simulink model "Homing_control"  (R2019b)
settings: Solver=FixedStepAuto  StartTime=0.0  StopTime=inf  FixedStep=0.01  RelTol=1e-3
undefined symbols (not defined in the file or in its folder): canChannel
libraries: canmsglib x13, simulink x7, canlib x3, sldrtlib x1
settings Model: Creator=Mohsen  LastModifiedBy=Mohsen
settings DataIOCC: ReturnWorkspaceOutputs=off
settings DebuggingCC: ArithmeticOperatorsInVariantConditions=warning
settings SFSimCC: SimUseLocalCustomCode=off  CustomCodeUndefinedFunction=UseInterfaceOnly
settings RTWCC: Description=Simulink Desktop Real-Time  SystemTargetFile=sldrt.tlc  TemplateMakefile=sldrt.tmf  RTWUseLocalCustomCode=off  RTWCompilerOptimization=on
settings CodeAppCC: MaxIdLength=95
settings TargetCC: TargetPreCompLibLocation=C:\Program Files\MATLAB\R2018b\toolbox\sldrt\lib\win64  TargetLangStandard=C99 (ISO)  GeneratePreprocessorConditionals=Use local settings  SupportVariableSizeSignals=on  PreserveStateflowLocalDataDimensions=off

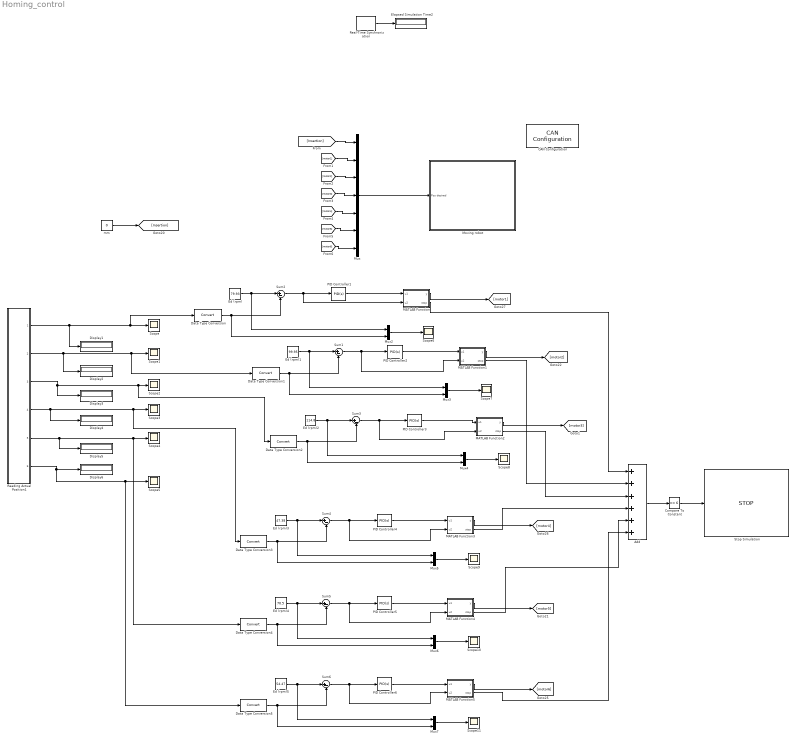
== system Homing_control ==
  Add : Sum  Inputs=++++++
  CAN Configuration : canlib/CAN Configuration  BlockHandle=3.0001  Device=Kvaser USBcan Light 1 (Channel 1)  DeviceMenu=Kvaser USBcan Light 1 (Channel 1)  ObjConstructor=canChannel('Kvaser', 'USBcan Light 1', 1)  BusSpeed=500000  EnableBitParameters=off  SJW=1  TSEG1=4  TSEG2=3  NSamples=1  AckMode=Normal
      settings: SourceProductName=Vehicle Network Toolbox  SourceProductBaseCode=VN
  Compare To Constant : simulink/Logic and Bit Operations/Compare To Constant  relop===  const=6  OutDataTypeStr=boolean
  Data Type Conversion{,1..5} (6 alike) : DataTypeConversion
  Display{1..6} (6 alike) : Display
  Ed (rpm) : Constant  Value=79.93
  Ed (rpm)1 : Constant  Value=99.95
  Ed (rpm)2 : Constant  Value=114.8
  Ed (rpm)3 : Constant  Value=47.38
  Ed (rpm)4 : Constant  Value=70.5
  Ed (rpm)5 : Constant  Value=54.47
  Elapsed Simulation Time2 : Display
      settings: Decimation=2
  MATLAB Function : MATLAB Function  TreatAsAtomicUnit=on
  MATLAB Function1 : MATLAB Function  TreatAsAtomicUnit=on
  MATLAB Function2 : MATLAB Function  TreatAsAtomicUnit=on
  MATLAB Function3 : MATLAB Function  TreatAsAtomicUnit=on
  MATLAB Function4 : MATLAB Function  TreatAsAtomicUnit=on
  MATLAB Function5 : MATLAB Function  TreatAsAtomicUnit=on
  Moving robot : Subsystem
  Mux : Mux  Inputs=7
  Mux{2..7} (6 alike) : Mux  Inputs=2
  PID Controller{1..6} (6 alike) : simulink/Continuous/PID Controller  Controller=PID  Form=Parallel  TimeDomain=Continuous-time  SampleTime=-1  IntegratorMethod=Forward Euler  FilterMethod=Forward Euler  ControllerParametersSource=internal  P=200  I=5  D=1  UseFilter=on  N=100  TunerSelectOption=Frequency Response Based  InitialConditionSource=internal  InitialConditionForIntegrator=0  InitialConditionForFilter=0  DifferentiatorICPrevScaledInput=0  ExternalReset=none  TrackingMode=off  Kt=1  LimitOutput=off  UpperSaturationLimit=inf  LowerSaturationLimit=-inf  LinearizeAsGain=on  AntiWindupMode=none  Kb=1  POutMin=[]  POutMax=[]  IOutMin=[]  IOutMax=[]  DOutMin=[]  DOutMax=[]  NOutMin=[]  NOutMax=[]  SumOutMin=[]  SumOutMax=[]  SaturationOutMin=[]  SaturationOutMax=[]  PParamMin=[]  PParamMax=[]  IParamMin=[]  IParamMax=[]  DParamMin=[]  DParamMax=[]  NParamMin=[]  NParamMax=[]  KbParamMin=[]  KbParamMax=[]  KtParamMin=[]  KtParamMax=[]  KbOutMin=[]  KbOutMax=[]  KtOutMin=[]  KtOutMax=[]  IntegratorOutMin=[]  IntegratorOutMax=[]  FilterOutMin=[]  FilterOutMax=[]  SumI1OutMin=[]  SumI1OutMax=[]  SumI2OutMin=[]  SumI2OutMax=[]  SumI3OutMin=[]  SumI3OutMax=[]  SumI4OutMin=[]  SumI4OutMax=[]  SumDOutMin=[]  SumDOutMax=[]  DifferentiatorOutMin=[]  DifferentiatorOutMax=[]  FilterDiffOutCoefMin=[]  FilterDiffOutCoefMax=[]  ReciprocalOutMin=[]  ReciprocalOutMax=[]  SumDenOutMin=[]  SumDenOutMax=[]  SumNumOutMin=[]  SumNumOutMax=[]  DivideOutMin=[]  DivideOutMax=[]  IntegratorContinuousStateAttributes=''  IntegratorStateMustResolveToSignalObject=off  IntegratorRTWStateStorageClass=Auto  FilterContinuousStateAttributes=''  FilterStateMustResolveToSignalObject=off  FilterRTWStateStorageClass=Auto  ParallelPVariant=InternalParameters  IdealPVariant=Disabled  IVariant=InternalParameters  DVariant=InternalParameters  IntegratorVariant=Continuous  SatVariant=Disabled  AWVariant=Passthrough  PCopyVariant=Disabled  TRVariant=Disabled  FdbkBlocksVariant=Forward  IdealPFdbkVariant=Disabled  SatFdbkVariant=Disabled  DerivativeFilterVariant=ContFilter  NVariant=InternalParameters  NCopyVariant=Disabled  FilterICVariant=InternalICsFilter  IntegratorICVariant=InternalICs  ExternalResetVariant=Disabled  TRSumVariant=Passthrough  SumFdbkVariant=Disabled  SumVariant=Sum_PID
  Reading Actual Position1 : Subsystem
  Real-Time Synchronization : sldrtlib/Real-Time Synchronization  SampleTime=-1  MaxMissedTicks=inf  ShowMissedTicks=on  YieldWhenWaiting=off
  Scope{,1..11} (12 alike) : Scope
  Stop Simulation : Stop
  Sum{1..6} (6 alike) : Sum  Inputs=|+-
  mm : Constant  Value=0
  wires:
  Mux/1 -> Moving robot/1(Pos desired)
  [motor6] -> Mux/7
  [motor5] -> Mux/6
  [motor4] -> Mux/5
  [motor3] -> Mux/4
  [motor2] -> Mux/3
  [motor1] -> Mux/2
  [Insertion] -> Mux/1
  mm/1 -> [Insertion]
  Real-Time Synchronization/1 -> Elapsed Simulation Time2/1
  Ed (rpm)/1 -> Mux2/1, Sum2/1
  Sum2/1 -> MATLAB Function/2(u2), PID Controller1/1
  Mux2/1 -> Scope6/1
  Reading Actual Position1/1(1) -> Data Type Conversion/1, Scope/1, Display1/1
  Data Type Conversion/1 -> Mux2/2, Sum2/2
  PID Controller1/1 -> MATLAB Function/1(u1)
  MATLAB Function1/1(y) -> [motor2]
  Mux3/1 -> Scope7/1
  Ed (rpm)1/1 -> Mux3/1, Sum1/1
  Reading Actual Position1/2(2) -> Display2/1, Data Type Conversion1/1, Scope1/1
  Sum1/1 -> PID Controller2/1, MATLAB Function1/2(u2)
  Data Type Conversion1/1 -> Mux3/2, Sum1/2
  PID Controller2/1 -> MATLAB Function1/1(u1)
  MATLAB Function2/1(y) -> [motor3]
  Mux4/1 -> Scope8/1
  Ed (rpm)2/1 -> Mux4/1, Sum3/1
  Reading Actual Position1/3(3) -> Data Type Conversion2/1, Scope2/1, Display3/1
  Sum3/1 -> MATLAB Function2/2(u2), PID Controller3/1
  Data Type Conversion2/1 -> Mux4/2, Sum3/2
  PID Controller3/1 -> MATLAB Function2/1(u1)
  MATLAB Function3/1(y) -> [motor4]
  Mux5/1 -> Scope9/1
  Ed (rpm)3/1 -> Mux5/1, Sum4/1
  Reading Actual Position1/4(4) -> Data Type Conversion3/1, Scope3/1, Display4/1
  Sum4/1 -> MATLAB Function3/2(u2), PID Controller4/1
  Data Type Conversion3/1 -> Mux5/2, Sum4/2
  PID Controller4/1 -> MATLAB Function3/1(u1)
  MATLAB Function4/1(y) -> [motor5]
  Mux6/1 -> Scope10/1
  Ed (rpm)4/1 -> Mux6/1, Sum5/1
  Reading Actual Position1/5(5) -> Display5/1, Data Type Conversion4/1, Scope4/1
  Sum5/1 -> MATLAB Function4/2(u2), PID Controller5/1
  Data Type Conversion4/1 -> Mux6/2, Sum5/2
  PID Controller5/1 -> MATLAB Function4/1(u1)
  MATLAB Function5/1(y) -> [motor6]
  Mux7/1 -> Scope11/1
  Ed (rpm)5/1 -> Mux7/1, Sum6/1
  Reading Actual Position1/6(6) -> Data Type Conversion5/1, Scope5/1, Display6/1
  Sum6/1 -> MATLAB Function5/2(u2), PID Controller6/1
  Data Type Conversion5/1 -> Mux7/2, Sum6/2
  PID Controller6/1 -> MATLAB Function5/1(u1)
  MATLAB Function/1(y) -> [motor1]
  Add/1 -> Compare To Constant/1
  MATLAB Function/2(stop) -> Add/1
  MATLAB Function1/2(stop) -> Add/2
  MATLAB Function2/2(stop) -> Add/3
  MATLAB Function3/2(stop) -> Add/4
  MATLAB Function4/2(stop) -> Add/5
  MATLAB Function5/2(stop) -> Add/6
  Compare To Constant/1 -> Stop Simulation/1

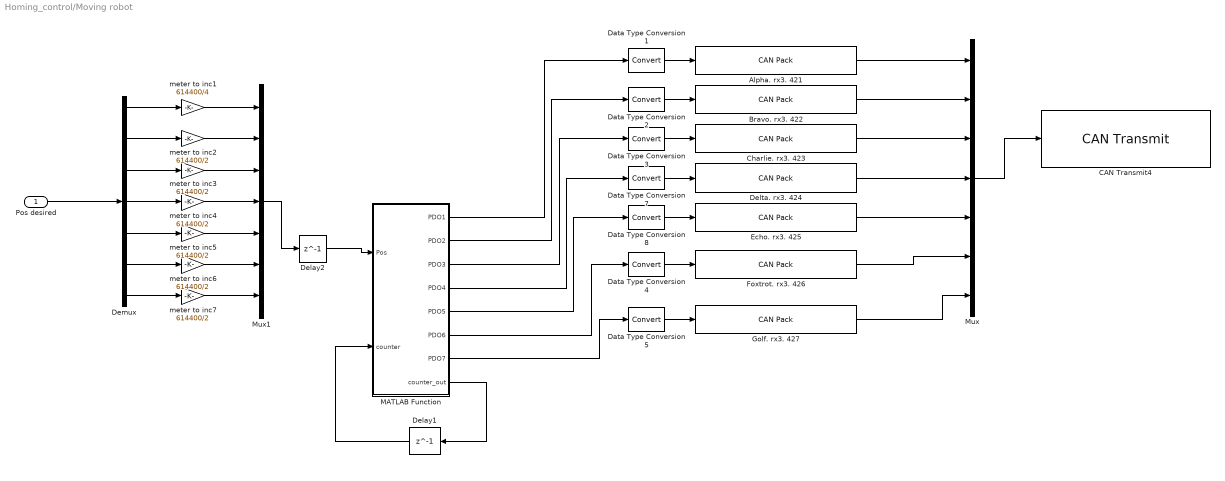
== system Homing_control/Moving robot ==
  Pos desired : Inport
  Alpha. rx3. 421 : canmsglib/CAN Pack  MsgList=(none)  MsgName=Alpha  MsgIDType=Standard (11-bit identifier)  MsgIdentifier=1057  MsgLength=8  Remote=off  ApplyMinMax=off  BusOutput=off  SignalInfo={ 'clear', '0', '64', 'LE', 'unsigned', 'Standard', '0', '1', '0', '-Inf', 'Inf' }
      settings: SourceProductName=Simulink Real-Time  SourceProductBaseCode=XP  DataFormat=raw data
  Bravo. rx3. 422 : canmsglib/CAN Pack  MsgList=(none)  MsgName=Bravo  MsgIDType=Standard (11-bit identifier)  MsgIdentifier=1058  MsgLength=8  Remote=off  ApplyMinMax=off  BusOutput=off  SignalInfo={ 'clear', '0', '64', 'LE', 'unsigned', 'Standard', '0', '1', '0', '-Inf', 'Inf' }
      settings: SourceProductName=Simulink Real-Time  SourceProductBaseCode=XP  DataFormat=raw data
  CAN Transmit4 : canlib/CAN Transmit  BlockHandle=1540.0004  Device=Kvaser USBcan Light 1 (Channel 1)  DeviceMenu=Kvaser USBcan Light 1 (Channel 1)  ObjConstructor=canChannel('Kvaser', 'USBcan Light 1', 1)  EnablePeriodicTransmit=off  MessagePeriod=0.500
      settings: SourceProductName=Vehicle Network Toolbox  SourceProductBaseCode=VN
  Charlie. rx3. 423 : canmsglib/CAN Pack  MsgList=(none)  MsgName=Charlie  MsgIDType=Standard (11-bit identifier)  MsgIdentifier=1059  MsgLength=8  Remote=off  ApplyMinMax=off  BusOutput=off  SignalInfo={ 'clear', '0', '64', 'LE', 'unsigned', 'Standard', '0', '1', '0', '-Inf', 'Inf' }
      settings: SourceProductName=Simulink Real-Time  SourceProductBaseCode=XP  DataFormat=raw data
  Data Type Conversion{1..5,7..8} (7 alike) : DataTypeConversion
  Delay1 : Delay  DelayLength=1  InitialCondition=0
  Delay2 : Delay  DelayLength=1  InitialCondition=[ 0 0 0 0 0 0 0]
  Delta. rx3. 424 : canmsglib/CAN Pack  MsgList=(none)  MsgName=Delta  MsgIDType=Standard (11-bit identifier)  MsgIdentifier=1060  MsgLength=8  Remote=off  ApplyMinMax=off  BusOutput=off  SignalInfo={ 'clear', '0', '64', 'LE', 'unsigned', 'Standard', '0', '1', '0', '-Inf', 'Inf' }
      settings: SourceProductName=Simulink Real-Time  SourceProductBaseCode=XP  DataFormat=raw data
  Demux : Demux  Outputs=7
  Echo. rx3. 425 : canmsglib/CAN Pack  MsgList=(none)  MsgName=Echo  MsgIDType=Standard (11-bit identifier)  MsgIdentifier=1061  MsgLength=8  Remote=off  ApplyMinMax=off  BusOutput=off  SignalInfo={ 'clear', '0', '64', 'LE', 'unsigned', 'Standard', '0', '1', '0', '-Inf', 'Inf' }
      settings: SourceProductName=Simulink Real-Time  SourceProductBaseCode=XP  DataFormat=raw data
  Foxtrot. rx3. 426 : canmsglib/CAN Pack  MsgList=(none)  MsgName=Foxtrot  MsgIDType=Standard (11-bit identifier)  MsgIdentifier=1062  MsgLength=8  Remote=off  ApplyMinMax=off  BusOutput=off  SignalInfo={ 'clear', '0', '64', 'LE', 'unsigned', 'Standard', '0', '1', '0', '-Inf', 'Inf' }
      settings: SourceProductName=Simulink Real-Time  SourceProductBaseCode=XP  DataFormat=raw data
  Golf. rx3. 427 : canmsglib/CAN Pack  MsgList=(none)  MsgName=Golf  MsgIDType=Standard (11-bit identifier)  MsgIdentifier=1063  MsgLength=8  Remote=off  ApplyMinMax=off  BusOutput=off  SignalInfo={ 'clear', '0', '64', 'LE', 'unsigned', 'Standard', '0', '1', '0', '-Inf', 'Inf' }
      settings: SourceProductName=Simulink Real-Time  SourceProductBaseCode=XP  DataFormat=raw data
  MATLAB Function : MATLAB Function  TreatAsAtomicUnit=on
  Mux : Mux  Inputs=7
  Mux1 : Mux  Inputs=7
  meter to inc1 : Gain  Gain=614400/4
  meter to inc{2..7} (6 alike) : Gain  Gain=614400/2
  wires:
  Data Type Conversion1/1 -> Alpha. rx3. 421/1
  MATLAB Function/8(counter_out) -> Delay1/1
  Delay1/1 -> MATLAB Function/2(counter)
  Mux/1 -> CAN Transmit4/1
  Mux1/1 -> Delay2/1
  Delay2/1 -> MATLAB Function/1(Pos)
  Alpha. rx3. 421/1 -> Mux/1
  Pos desired/1 -> Demux/1
  Demux/7 -> meter to inc7/1
  meter to inc7/1 -> Mux1/7
  Demux/6 -> meter to inc6/1
  meter to inc6/1 -> Mux1/6
  meter to inc5/1 -> Mux1/5
  Demux/5 -> meter to inc5/1
  Demux/4 -> meter to inc4/1
  meter to inc4/1 -> Mux1/4
  meter to inc3/1 -> Mux1/3
  meter to inc2/1 -> Mux1/2
  meter to inc1/1 -> Mux1/1
  Demux/1 -> meter to inc1/1
  Demux/2 -> meter to inc2/1
  Demux/3 -> meter to inc3/1
  Data Type Conversion2/1 -> Bravo. rx3. 422/1
  Data Type Conversion3/1 -> Charlie. rx3. 423/1
  Data Type Conversion7/1 -> Delta. rx3. 424/1
  Data Type Conversion8/1 -> Echo. rx3. 425/1
  Bravo. rx3. 422/1 -> Mux/2
  Charlie. rx3. 423/1 -> Mux/3
  Delta. rx3. 424/1 -> Mux/4
  Echo. rx3. 425/1 -> Mux/5
  MATLAB Function/1(PDO1) -> Data Type Conversion1/1
  MATLAB Function/2(PDO2) -> Data Type Conversion2/1
  MATLAB Function/3(PDO3) -> Data Type Conversion3/1
  MATLAB Function/4(PDO4) -> Data Type Conversion7/1
  MATLAB Function/5(PDO5) -> Data Type Conversion8/1
  Data Type Conversion4/1 -> Foxtrot. rx3. 426/1
  Data Type Conversion5/1 -> Golf. rx3. 427/1
  MATLAB Function/6(PDO6) -> Data Type Conversion4/1
  MATLAB Function/7(PDO7) -> Data Type Conversion5/1
  Foxtrot. rx3. 426/1 -> Mux/6
  Golf. rx3. 427/1 -> Mux/7

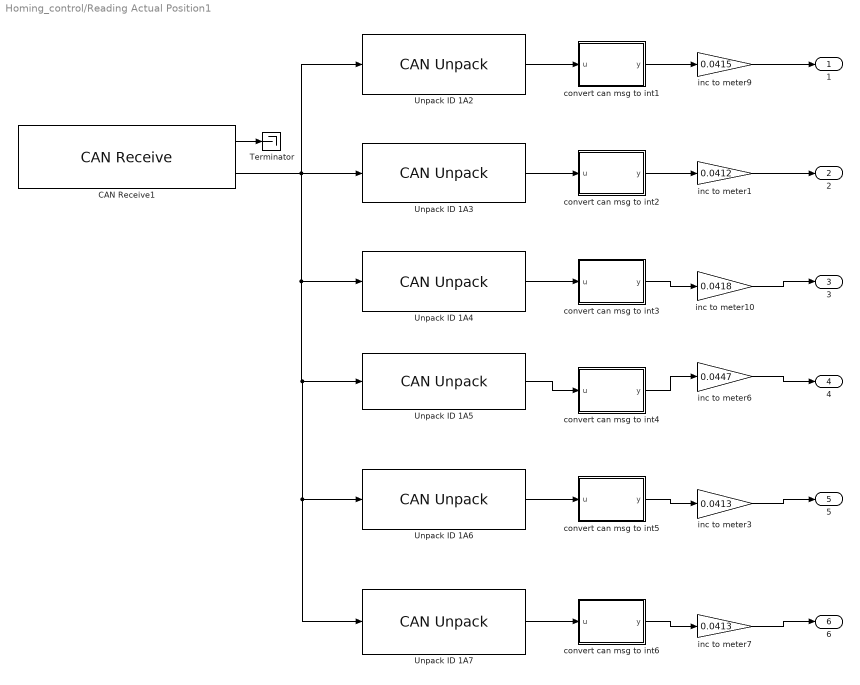
== system Homing_control/Reading Actual Position1 ==
  CAN Receive1 : canlib/CAN Receive  BlockHandle=1635.0002  Device=Kvaser USBcan Light 1 (Channel 1)  DeviceMenu=Kvaser USBcan Light 1 (Channel 1)  ObjConstructor=canChannel('Kvaser', 'USBcan Light 1', 1)  EnableStandardIDsFilter=off  StdIDsCombo=Allow only  StandardIDs=[418 419 420 421 422 423]  EnableExtendedIDsFilter=off  ExtIDsCombo=Allow all  ExtendedIDs=0  SampleTime=-1  MsgsPerTimestep=all  InternalFilterUpdateStatus=on  BusOutput=off
      settings: SourceProductName=Vehicle Network Toolbox  SourceProductBaseCode=VN
  Terminator : Terminator
  Unpack ID 1A2 : canmsglib/CAN Unpack  MsgList=(none)  MsgName=CAN Msg  MsgIDType=Standard (11-bit identifier)  MsgIdentifier=418  MsgLength=2  SignalInfo={ 'Counter', '8', '16', 'LE', 'unsigned', 'Standard', '0', '1', '0', '-Inf', 'Inf' }  IDPort=off  TimestampPort=off  ErrorPort=off  RemotePort=off  LengthPort=off  StatusPort=off  ApplyMinMax=off
      settings: SourceProductName=Simulink Real-Time  SourceProductBaseCode=XP  DataFormat=raw data
  Unpack ID 1A3 : canmsglib/CAN Unpack  MsgList=(none)  MsgName=CAN Msg  MsgIDType=Standard (11-bit identifier)  MsgIdentifier=419  MsgLength=2  SignalInfo={ 'Counter', '8', '16', 'LE', 'unsigned', 'Standard', '0', '1', '0', '-Inf', 'Inf' }  IDPort=off  TimestampPort=off  ErrorPort=off  RemotePort=off  LengthPort=off  StatusPort=off  ApplyMinMax=off
      settings: SourceProductName=Simulink Real-Time  SourceProductBaseCode=XP  DataFormat=raw data
  Unpack ID 1A4 : canmsglib/CAN Unpack  MsgList=(none)  MsgName=CAN Msg  MsgIDType=Standard (11-bit identifier)  MsgIdentifier=420  MsgLength=2  SignalInfo={ 'Counter', '8', '16', 'LE', 'unsigned', 'Standard', '0', '1', '0', '-Inf', 'Inf' }  IDPort=off  TimestampPort=off  ErrorPort=off  RemotePort=off  LengthPort=off  StatusPort=off  ApplyMinMax=off
      settings: SourceProductName=Simulink Real-Time  SourceProductBaseCode=XP  DataFormat=raw data
  Unpack ID 1A5 : canmsglib/CAN Unpack  MsgList=(none)  MsgName=CAN Msg  MsgIDType=Standard (11-bit identifier)  MsgIdentifier=421  MsgLength=2  SignalInfo={ 'Counter', '8', '16', 'LE', 'unsigned', 'Standard', '0', '1', '0', '-Inf', 'Inf' }  IDPort=off  TimestampPort=off  ErrorPort=off  RemotePort=off  LengthPort=off  StatusPort=off  ApplyMinMax=off
      settings: SourceProductName=Simulink Real-Time  SourceProductBaseCode=XP  DataFormat=raw data
  Unpack ID 1A6 : canmsglib/CAN Unpack  MsgList=(none)  MsgName=CAN Msg  MsgIDType=Standard (11-bit identifier)  MsgIdentifier=422  MsgLength=2  SignalInfo={ 'Counter', '8', '16', 'LE', 'unsigned', 'Standard', '0', '1', '0', '-Inf', 'Inf' }  IDPort=off  TimestampPort=off  ErrorPort=off  RemotePort=off  LengthPort=off  StatusPort=off  ApplyMinMax=off
      settings: SourceProductName=Simulink Real-Time  SourceProductBaseCode=XP  DataFormat=raw data
  Unpack ID 1A7 : canmsglib/CAN Unpack  MsgList=(none)  MsgName=CAN Msg  MsgIDType=Standard (11-bit identifier)  MsgIdentifier=423  MsgLength=2  SignalInfo={ 'Counter', '8', '16', 'LE', 'unsigned', 'Standard', '0', '1', '0', '-Inf', 'Inf' }  IDPort=off  TimestampPort=off  ErrorPort=off  RemotePort=off  LengthPort=off  StatusPort=off  ApplyMinMax=off
      settings: SourceProductName=Simulink Real-Time  SourceProductBaseCode=XP  DataFormat=raw data
  convert can msg to int1 : MATLAB Function  TreatAsAtomicUnit=on
  convert can msg to int2 : MATLAB Function  TreatAsAtomicUnit=on
  convert can msg to int3 : MATLAB Function  TreatAsAtomicUnit=on
  convert can msg to int4 : MATLAB Function  TreatAsAtomicUnit=on
  convert can msg to int5 : MATLAB Function  TreatAsAtomicUnit=on
  convert can msg to int6 : MATLAB Function  TreatAsAtomicUnit=on
  inc to meter1 : Gain  Gain=0.0412
  inc to meter10 : Gain  Gain=0.0418
  inc to meter3 : Gain  Gain=0.0413
  inc to meter6 : Gain  Gain=0.0447
  inc to meter7 : Gain  Gain=0.0413
  inc to meter9 : Gain  Gain=0.0415
  1 : Outport  VectorParamsAs1DForOutWhenUnconnected=off
  2 : Outport  Port=2  VectorParamsAs1DForOutWhenUnconnected=off
  3 : Outport  Port=3  VectorParamsAs1DForOutWhenUnconnected=off
  4 : Outport  Port=4  VectorParamsAs1DForOutWhenUnconnected=off
  5 : Outport  Port=5  VectorParamsAs1DForOutWhenUnconnected=off
  6 : Outport  Port=6  VectorParamsAs1DForOutWhenUnconnected=off
  wires:
  convert can msg to int3/1(y) -> inc to meter10/1
  inc to meter10/1 -> 3/1
  convert can msg to int2/1(y) -> inc to meter1/1
  Unpack ID 1A3/1 -> convert can msg to int2/1(u)
  Unpack ID 1A5/1 -> convert can msg to int4/1(u)
  inc to meter1/1 -> 2/1
  convert can msg to int5/1(y) -> inc to meter3/1
  inc to meter3/1 -> 5/1
  Unpack ID 1A7/1 -> convert can msg to int6/1(u)
  inc to meter7/1 -> 6/1
  Unpack ID 1A6/1 -> convert can msg to int5/1(u)
  Unpack ID 1A4/1 -> convert can msg to int3/1(u)
  convert can msg to int6/1(y) -> inc to meter7/1
  CAN Receive1/1 -> Terminator/1
  inc to meter6/1 -> 4/1
  convert can msg to int4/1(y) -> inc to meter6/1
  CAN Receive1/2 -> Unpack ID 1A7/1, Unpack ID 1A6/1, Unpack ID 1A5/1, Unpack ID 1A4/1, Unpack ID 1A2/1, Unpack ID 1A3/1
  Unpack ID 1A2/1 -> convert can msg to int1/1(u)
  inc to meter9/1 -> 1/1
  convert can msg to int1/1(y) -> inc to meter9/1

== matlab function Homing_control/Moving robot/MATLAB Function ==
  data: PDO1 output; PDO2 output; PDO3 output; PDO4 output; PDO5 output; PDO6 output; PDO7 output; Pos input; counter input; counter_out output
function [PDO1,PDO2,PDO3,PDO4,PDO5,PDO6,PDO7,counter_out]   = fcn(Pos,counter)

%Initializing outputs
PDO=zeros(10,6); counter_out=counter;


if counter==1 % send pos signal
    for i=1:7
        p =dec2hex(swapbytes(typecast(int32(Pos(i)),'uint32')),8);
        PDO(i,:)=[hex2dec('3F') hex2dec('00') hex2dec(p(1:2)) hex2dec(p(3:4)) hex2dec(p(5:6)) hex2dec(p(7:8))];
    end
    counter_out=0;
elseif counter==0 % activate pos signal  
    for i=1:7
        PDO(i,:)=[hex2dec('0F') hex2dec('00') 0 0 0 0]; 
    end
    counter_out=1;
end

PDO1=PDO(1,:);
PDO2=PDO(2,:);
PDO3=PDO(3,:);
PDO4=PDO(4,:);
PDO5=PDO(5,:);
PDO6=PDO(6,:);
PDO7=PDO(7,:);
end

== matlab function Homing_control/MATLAB Function ==
  data: u1 input; y output; u2 input; stop output
function [y, stop]= fcn(u1,u2)

if abs(u2)>=0.5
    y = u1;
    stop=0
else
    y = 0;
    stop=1
end

== matlab function Homing_control/MATLAB Function1 ==
  data: u1 input; y output; u2 input; stop output
function [y, stop]= fcn(u1,u2)

if abs(u2)>=0.5
    y = u1;
    stop=0
else
    y = 0;
    stop=1
end

== matlab function Homing_control/MATLAB Function2 ==
  data: u1 input; y output; u2 input; stop output
function [y, stop]= fcn(u1,u2)

if abs(u2)>=0.5
    y = u1;
    stop=0
else
    y = 0;
    stop=1
end

== matlab function Homing_control/MATLAB Function3 ==
  data: u1 input; y output; u2 input; stop output
function [y, stop]= fcn(u1,u2)

if abs(u2)>=0.5
    y = u1;
    stop=0
else
    y = 0;
    stop=1
end

== matlab function Homing_control/MATLAB Function4 ==
  data: u1 input; y output; u2 input; stop output
function [y, stop]= fcn(u1,u2)

if abs(u2)>=0.5
    y = u1;
    stop=0
else
    y = 0;
    stop=1
end

== matlab function Homing_control/MATLAB Function5 ==
  data: u1 input; y output; u2 input; stop output
function [y, stop]= fcn(u1,u2)

if abs(u2)>=0.5
    y = u1;
    stop=0
else
    y = 0;
    stop=1
end

== matlab function Homing_control/Reading Actual Position1/convert can msg to int1 ==
  data: u input; y output
function y = fcn(u)
y = int32(0);
msg=[dec2hex(u(2),2) dec2hex(u(1),2)];
y=typecast(uint32(hex2dec(msg)),'int32');

== matlab function Homing_control/Reading Actual Position1/convert can msg to int2 ==
  data: u input; y output
function y = fcn(u)
y = int32(0);
msg=[dec2hex(u(2),2) dec2hex(u(1),2)];
y=typecast(uint32(hex2dec(msg)),'int32');

== matlab function Homing_control/Reading Actual Position1/convert can msg to int3 ==
  data: u input; y output
function y = fcn(u)
y = int32(0);
msg=[dec2hex(u(2),2) dec2hex(u(1),2)];
y=typecast(uint32(hex2dec(msg)),'int32');

== matlab function Homing_control/Reading Actual Position1/convert can msg to int4 ==
  data: u input; y output
function y = fcn(u)
y = int32(0);
msg=[dec2hex(u(2),2) dec2hex(u(1),2)];
y=typecast(uint32(hex2dec(msg)),'int32');

== matlab function Homing_control/Reading Actual Position1/convert can msg to int5 ==
  data: u input; y output
function y = fcn(u)
y = int32(0);
msg=[dec2hex(u(2),2) dec2hex(u(1),2)];
y=typecast(uint32(hex2dec(msg)),'int32');

== matlab function Homing_control/Reading Actual Position1/convert can msg to int6 ==
  data: u input; y output
function y = fcn(u)
y = int32(0);
msg=[dec2hex(u(2),2) dec2hex(u(1),2)];
y=typecast(uint32(hex2dec(msg)),'int32');
